simulink model "EST"  (R2026a)
settings: Solver=FixedStepAuto  StopTime=stopt  FixedStep=deltat  MaxStep=0.05
InitFcn:
  | clear all;
  | close all;
  | clc;
  | 
  | % add the data and script directories
  | addpath('data','scripts');
  | 
  | % load the constants (units)
  | constants;
  | 
  | % load the simulation parameters
  | preprocessing;
StopFcn:
  | postprocessing;
values from neighbouring files (symbols this model uses):
  alphaLoss = 0.15    [preprocessing.m]
  alphaSplit = 0.7    [preprocessing.m]
  areaTank = 6 * sideLength^2    (= 57.9293630763)    [preprocessing.m]
  cableArea = 6e-6    (= 6e-06)    [preprocessing.m]
  cableLength = 28.5    [preprocessing.m]
  cableLengthDemand = 20    [preprocessing.m]
  cableResistivity = 1.676e-8    (= 1.676e-08)    [preprocessing.m]
  cps = 920    [preprocessing.m]
  current = 20    [preprocessing.m]
  currentDemand = 2.5    [preprocessing.m]
  dh_ads = 2.5e6    (= 2500000)    [preprocessing.m]
  dtController = 900    [preprocessing.m]
  E = E_DA    (= 6000)    [preprocessing.m]
  EBatteryMax = 200 * 3.6e6    (= 720000000)    [preprocessing.m]
  EBatteryMin = 0  * 3.6e6    (= 0)    [preprocessing.m]
  efficiencyBatteryCharge = 0.95    [preprocessing.m]
  efficiencyInjection = 0.98    [preprocessing.m]
  emissivitySurface = 0.5    [preprocessing.m]
  emissivitySurfacePipe = 0.9    [preprocessing.m]
  EStorageMax = 5000 * 3.6e6    (= 18000000000)    [preprocessing.m]
  EStorageMin = 100  * 3.6e6    (= 360000000)    [preprocessing.m]
  etaBatteryDischarge = 0.95    [preprocessing.m]
  hAir = 10    [preprocessing.m]
  kInsulation = 0.04    [preprocessing.m]
  kLdf = 0.008    [preprocessing.m]
  kPipe = 0.3    [preprocessing.m]
  kSteel = 54    [preprocessing.m]
  mCpTotal = massGel * heatCapacityGel + massSteel * heatCapacitySteel    (= 21486379.4261)    [preprocessing.m]
  ms = massGel    (= 21600)    [preprocessing.m]
  n = 1.5    [preprocessing.m]
  pipeLength = 10    [preprocessing.m]
  PmaxBatteryCharge = 20    [preprocessing.m]
  PmaxBatteryDischarge = 20    [preprocessing.m]
  PmaxSorptionCharge = 5    [preprocessing.m]
  PmaxSorptionDischarge = 15    [preprocessing.m]
  pv = 1200    [preprocessing.m]
  r1 = 0.03    [preprocessing.m]
  r2 = 0.035    [preprocessing.m]
  r3 = 0.05    [preprocessing.m]
  stefanBoltz = 5.67e-8    (= 5.67e-08)    [preprocessing.m]
  tempEnv = 293.15    [preprocessing.m]
  Tfluid = 353.15    [preprocessing.m]
  thicknessInsulation = 0.10    (= 0.1)    [preprocessing.m]
  thicknessSteel = 0.015    [preprocessing.m]
  Tref = tempEnv    (= 293.15)    [preprocessing.m]
  TStorageInitial = Tref    (= 293.15)    [preprocessing.m]
  UA = 15    [preprocessing.m]
  X0 = 0.35    [preprocessing.m]
  Xref = X0    (= 0.35)    [preprocessing.m]
  XStorageInitial = max(0.0, min(X0, XStorageInitial))    [preprocessing.m]
settings Model: Creator=joche  LastModifiedBy=nimaaminpour
settings SimscapeCC: SimscapeLogDataHistory=5000.0  SimscapeNominalValues="[{\"value\":\"1\",\"unit\":\"A\"},{\"value\":\"1\",\"unit\":\"bar\"},{\"value\":\"1\",\"unit\":\"cm^2\"},{\"value\":\"1\",\"unit\":\"cm^3/s\"},{\"value\":\"1\",\"unit\":\"kJ/kg\"},{\"value\":\"1\",\"unit\":\"kW\"},{\"value\":\"1\",\"unit\":\"l\"},{\"value\":\"1\",\"unit\":\"N\"},{\"value\":\"1\",\"unit\":\"N*m\"},{\"value\":\"1\",\"unit\":\"V\"}]"  SimscapeLogType=none

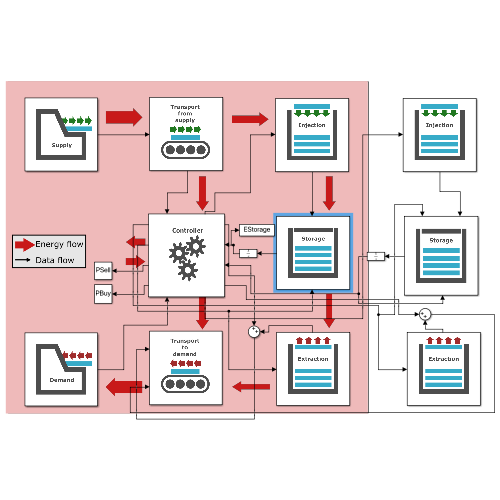
[thumbnail: Simulink's stored preview of the top-level diagram]
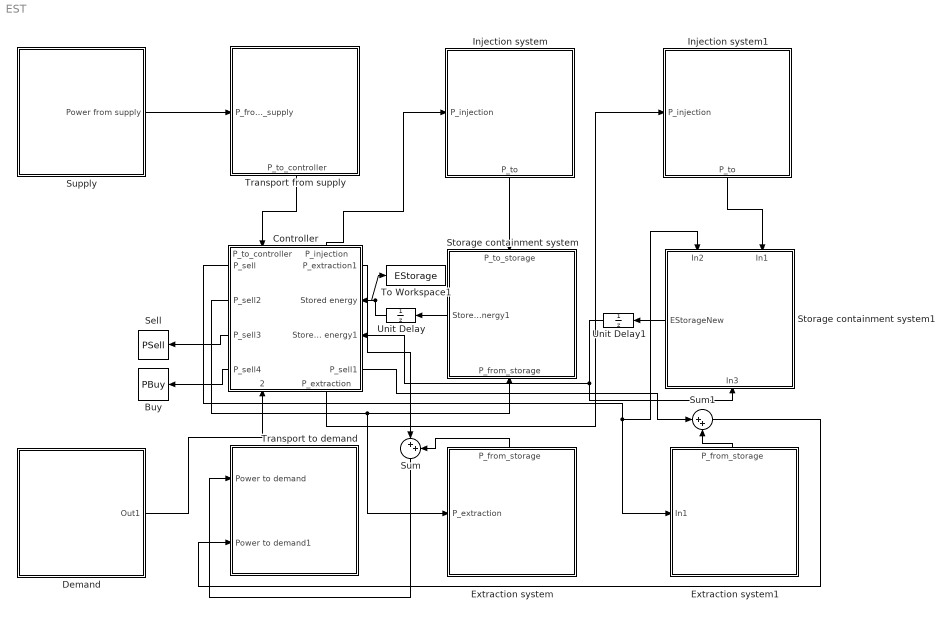
== system EST ==
  Buy : ToWorkspace  VariableName=PBuy  SampleTime=-1
  Controller : Subsystem
      settings: PortSchema="{\"entries\":[{\"content\":{\"sides\":[{\"content\":{\"connectorIds\":[\"Out5\",\"Out6\",\"Out7\",\"Out8\"]},\"type\":\"ConnectorPlacement.EquallySpacedRectSide\",\"uuid\":\"4daf33ce-c96a-4783-b5c4-228eed953e01\"},{\"content\":{\"connectorIds\":[\"Out1\",\"In3\",\"In4\",\"Out2\"],\"side\":\"RIGHT\"},\"type\":\"ConnectorPlacement.EquallySpacedRectSide\",\"uuid\":\"e9942e50-8467-4af8-b79b-80636cbc76e5\"},{\"content\":{\"connectorIds\":[\"In1\",\"Out4\"],\"side\":\"TOP\"},\"type\":\"ConnectorPlacement.EquallySpacedRectSide\",\"uuid\":\"f315e931-d69b-4751-b712-f89c6c81baeb\"},{\"content\":{\"connectorIds\":[\"In2\",\"Out3\"],\"side\":\"BOTTOM\"},\"type\":\"ConnectorPlacement.EquallySpacedRectSide\",\"uuid\":\"44715ee6-5cd5-4669-bcb9-5ed7c869bdb3\"}]},\"type\":\"ConnectorPlacement.EquallySpacedConnector\",\"uuid\":\"fff48899-944b-4064-b7d7-ecc12144fb48\"}],\"packageUris\":[\"http://schema.mathworks.com/mf0/Connector/R2020b\"],\"version\":\"1.0\"}"
      mask Display: image('$imagefile'); % Use "Edit Image" on toolstrip to change.
  Demand : Subsystem
      mask Display: image('$imagefile'); % Use "Edit Image" on toolstrip to change.
  Extraction system : Subsystem
      settings: PortSchema="{\"entries\":[{\"content\":{\"sides\":[{\"content\":{\"connectorIds\":[]},\"type\":\"ConnectorPlacement.EquallySpacedRectSide\",\"uuid\":\"05c5933d-55fc-4e06-853f-fc26d42905f9\"},{\"content\":{\"connectorIds\":[\"In1\"],\"side\":\"RIGHT\"},\"type\":\"ConnectorPlacement.EquallySpacedRectSide\",\"uuid\":\"327426c5-31d5-498b-a2bd-83e49353408c\"},{\"content\":{\"connectorIds\":[],\"side\":\"TOP\"},\"type\":\"ConnectorPlacement.EquallySpacedRectSide\",\"uuid\":\"55306cf3-a3de-4385-a5ae-b8600ecdd5a2\"},{\"content\":{\"connectorIds\":[\"Out1\"],\"side\":\"BOTTOM\"},\"type\":\"ConnectorPlacement.EquallySpacedRectSide\",\"uuid\":\"08fcc9c3-40d3-4ac6-b914-dfeef6039ffb\"}]},\"type\":\"ConnectorPlacement.EquallySpacedConnector\",\"uuid\":\"cb35d5ba-e8c6-462c-b7b2-fe8356d4b0a1\"}],\"packageUris\":[\"http://schema.mathworks.com/mf0/Connector/R2020b\"],\"version\":\"1.0\"}"
      mask Display: image('$imagefile'); % Use "Edit Image" on toolstrip to change.
  Extraction system1 : Subsystem
      settings: PortSchema="{\"entries\":[{\"content\":{\"sides\":[{\"content\":{},\"type\":\"ConnectorPlacement.EquallySpacedRectSide\",\"uuid\":\"05c5933d-55fc-4e06-853f-fc26d42905f9\"},{\"content\":{\"connectorIds\":[\"In1\"],\"side\":\"RIGHT\"},\"type\":\"ConnectorPlacement.EquallySpacedRectSide\",\"uuid\":\"327426c5-31d5-498b-a2bd-83e49353408c\"},{\"content\":{\"side\":\"TOP\"},\"type\":\"ConnectorPlacement.EquallySpacedRectSide\",\"uuid\":\"55306cf3-a3de-4385-a5ae-b8600ecdd5a2\"},{\"content\":{\"connectorIds\":[\"Out1\"],\"side\":\"BOTTOM\"},\"type\":\"ConnectorPlacement.EquallySpacedRectSide\",\"uuid\":\"08fcc9c3-40d3-4ac6-b914-dfeef6039ffb\"}]},\"type\":\"ConnectorPlacement.EquallySpacedConnector\",\"uuid\":\"cb35d5ba-e8c6-462c-b7b2-fe8356d4b0a1\"}],\"packageUris\":[\"http://schema.mathworks.com/mf0/Connector/R2020b\"],\"version\":\"1.0\"}"
      mask Display: image('$imagefile'); % Use "Edit Image" on toolstrip to change.
  Injection system : Subsystem
      settings: PortSchema="{\"entries\":[{\"content\":{\"sides\":[{\"content\":{\"connectorIds\":[]},\"type\":\"ConnectorPlacement.EquallySpacedRectSide\",\"uuid\":\"05c5933d-55fc-4e06-853f-fc26d42905f9\"},{\"content\":{\"connectorIds\":[\"In1\"],\"side\":\"RIGHT\"},\"type\":\"ConnectorPlacement.EquallySpacedRectSide\",\"uuid\":\"327426c5-31d5-498b-a2bd-83e49353408c\"},{\"content\":{\"connectorIds\":[\"Out1\"],\"side\":\"TOP\"},\"type\":\"ConnectorPlacement.EquallySpacedRectSide\",\"uuid\":\"55306cf3-a3de-4385-a5ae-b8600ecdd5a2\"},{\"content\":{\"connectorIds\":[],\"side\":\"BOTTOM\"},\"type\":\"ConnectorPlacement.EquallySpacedRectSide\",\"uuid\":\"08fcc9c3-40d3-4ac6-b914-dfeef6039ffb\"}]},\"type\":\"ConnectorPlacement.EquallySpacedConnector\",\"uuid\":\"cb35d5ba-e8c6-462c-b7b2-fe8356d4b0a1\"}],\"packageUris\":[\"http://schema.mathworks.com/mf0/Connector/R2020b\"],\"version\":\"1.0\"}"
      mask Display: image('$imagefile'); % Use "Edit Image" on toolstrip to change.
  Injection system1 : Subsystem
      settings: PortSchema="{\"entries\":[{\"content\":{\"sides\":[{\"content\":{\"connectorIds\":[]},\"type\":\"ConnectorPlacement.EquallySpacedRectSide\",\"uuid\":\"05c5933d-55fc-4e06-853f-fc26d42905f9\"},{\"content\":{\"connectorIds\":[\"In1\"],\"side\":\"RIGHT\"},\"type\":\"ConnectorPlacement.EquallySpacedRectSide\",\"uuid\":\"327426c5-31d5-498b-a2bd-83e49353408c\"},{\"content\":{\"connectorIds\":[\"Out1\"],\"side\":\"TOP\"},\"type\":\"ConnectorPlacement.EquallySpacedRectSide\",\"uuid\":\"55306cf3-a3de-4385-a5ae-b8600ecdd5a2\"},{\"content\":{\"connectorIds\":[],\"side\":\"BOTTOM\"},\"type\":\"ConnectorPlacement.EquallySpacedRectSide\",\"uuid\":\"08fcc9c3-40d3-4ac6-b914-dfeef6039ffb\"}]},\"type\":\"ConnectorPlacement.EquallySpacedConnector\",\"uuid\":\"cb35d5ba-e8c6-462c-b7b2-fe8356d4b0a1\"}],\"packageUris\":[\"http://schema.mathworks.com/mf0/Connector/R2020b\"],\"version\":\"1.0\"}"
      mask Display: image('$imagefile'); % Use "Edit Image" on toolstrip to change.
  Sell : ToWorkspace  VariableName=PSell  SampleTime=-1
  Storage containment system : Subsystem
      settings: PortSchema="{\"entries\":[{\"content\":{\"sides\":[{\"content\":{\"connectorIds\":[\"Out1\"]},\"type\":\"ConnectorPlacement.EquallySpacedRectSide\",\"uuid\":\"0ba48424-33b9-4934-970f-64fe5d8b070e\"},{\"content\":{\"connectorIds\":[],\"side\":\"RIGHT\"},\"type\":\"ConnectorPlacement.EquallySpacedRectSide\",\"uuid\":\"9cde340f-8f39-4499-9a12-5e1623737660\"},{\"content\":{\"connectorIds\":[\"In1\"],\"side\":\"TOP\"},\"type\":\"ConnectorPlacement.EquallySpacedRectSide\",\"uuid\":\"2af8db04-7fd0-4902-8637-8dc00edb4598\"},{\"content\":{\"connectorIds\":[\"In2\"],\"side\":\"BOTTOM\"},\"type\":\"ConnectorPlacement.EquallySpacedRectSide\",\"uuid\":\"e21ea806-d777-41a3-a53f-556fae66854b\"}]},\"type\":\"ConnectorPlacement.EquallySpacedConnector\",\"uuid\":\"4e2ddb36-4db3-4ab4-858b-ebb8ccefeb1f\"}],\"packageUris\":[\"http://schema.mathworks.com/mf0/Connector/R2020b\"],\"version\":\"1.0\"}"
      mask Display: image('$imagefile'); % Use "Edit Image" on toolstrip to change.
  Storage containment system1 : Subsystem
      settings: PortSchema="{\"entries\":[{\"content\":{\"sides\":[{\"content\":{\"connectorIds\":[\"Out1\"]},\"type\":\"ConnectorPlacement.EquallySpacedRectSide\",\"uuid\":\"0ba48424-33b9-4934-970f-64fe5d8b070e\"},{\"content\":{\"side\":\"RIGHT\"},\"type\":\"ConnectorPlacement.EquallySpacedRectSide\",\"uuid\":\"9cde340f-8f39-4499-9a12-5e1623737660\"},{\"content\":{\"connectorIds\":[\"In1\",\"In2\"],\"side\":\"TOP\"},\"type\":\"ConnectorPlacement.EquallySpacedRectSide\",\"uuid\":\"2af8db04-7fd0-4902-8637-8dc00edb4598\"},{\"content\":{\"connectorIds\":[\"In3\"],\"side\":\"BOTTOM\"},\"type\":\"ConnectorPlacement.EquallySpacedRectSide\",\"uuid\":\"e21ea806-d777-41a3-a53f-556fae66854b\"}]},\"type\":\"ConnectorPlacement.EquallySpacedConnector\",\"uuid\":\"4e2ddb36-4db3-4ab4-858b-ebb8ccefeb1f\"}],\"packageUris\":[\"http://schema.mathworks.com/mf0/Connector/R2020b\"],\"version\":\"1.0\"}"
      mask Display: image('$imagefile'); % Use "Edit Image" on toolstrip to change.
  Sum : Sum  Inputs=|++
  Sum1 : Sum  Inputs=|++
  Supply : Subsystem
      mask Display: image('$imagefile'); % Use "Edit Image" on toolstrip to change.
  To Workspace1 : ToWorkspace  VariableName=EStorage  SampleTime=-1
  Transport from supply : Subsystem
      settings: PortSchema="{\"entries\":[{\"content\":{\"sides\":[{\"content\":{\"connectorIds\":[\"In1\"]},\"type\":\"ConnectorPlacement.EquallySpacedRectSide\",\"uuid\":\"31329006-3d36-4d93-9c44-7503a515d397\"},{\"content\":{\"connectorIds\":[],\"side\":\"RIGHT\"},\"type\":\"ConnectorPlacement.EquallySpacedRectSide\",\"uuid\":\"aba139c7-f9b6-4881-a56b-a4cbbedacd88\"},{\"content\":{\"connectorIds\":[],\"side\":\"TOP\"},\"type\":\"ConnectorPlacement.EquallySpacedRectSide\",\"uuid\":\"e683eb73-7a35-4160-9c39-da83856a6278\"},{\"content\":{\"connectorIds\":[\"Out1\"],\"side\":\"BOTTOM\"},\"type\":\"ConnectorPlacement.EquallySpacedRectSide\",\"uuid\":\"1170dd18-447c-437f-9043-6812c2877331\"}]},\"type\":\"ConnectorPlacement.EquallySpacedConnector\",\"uuid\":\"804af608-1d70-444f-af69-e05f19bf98f3\"}],\"packageUris\":[\"http://schema.mathworks.com/mf0/Connector/R2020b\"],\"version\":\"1.0\"}"
      mask Display: image('$imagefile'); % Use "Edit Image" on toolstrip to change.
  Transport to demand : Subsystem
      mask Display: image('$imagefile'); % Use "Edit Image" on toolstrip to change.
  Unit Delay : UnitDelay  SampleTime=-1
  Unit Delay1 : UnitDelay  SampleTime=-1
  wires:
  Supply/1(Power from supply) -> Transport from supply/1(P_from_supply)
  Transport from supply/1(P_to_controller) -> Controller/1(P_to_controller)
  Injection system/1(P_to) -> Storage containment system/1(P_to_storage)
  Storage containment system/1(Stored energy1) -> Unit Delay/1
  Controller/8(P_sell4) -> Buy/1
  Injection system1/1(P_to) -> Storage containment system1/2(In1)
  Storage containment system1/1(EStorageNew) -> Unit Delay1/1
  Demand/1(Out1) -> Controller/2(P_from_controller)
  Unit Delay/1 -> To Workspace1/1, Controller/3(Stored energy)
  Unit Delay1/1 -> Storage containment system1/3(In3), Controller/4(Stored energy1)
  Controller/7(P_sell3) -> Sell/1
  Controller/5(P_sell) -> Storage containment system1/1(In2), Extraction system1/1(In1)
  Controller/6(P_sell2) -> Storage containment system/2(P_from_storage), Extraction system/1(P_extraction)
  Controller/1(P_extraction1) -> Sum/1
  Extraction system/1(P_from_storage) -> Sum/2
  Controller/2(P_sell1) -> Sum1/1
  Extraction system1/1(P_from_storage) -> Sum1/2
  Sum/1 -> Transport to demand/1(Power to demand)
  Sum1/1 -> Transport to demand/2(Power to demand1)
  Controller/3(P_extraction) -> Injection system1/1(P_injection)
  Controller/4(P_injection) -> Injection system/1(P_injection)

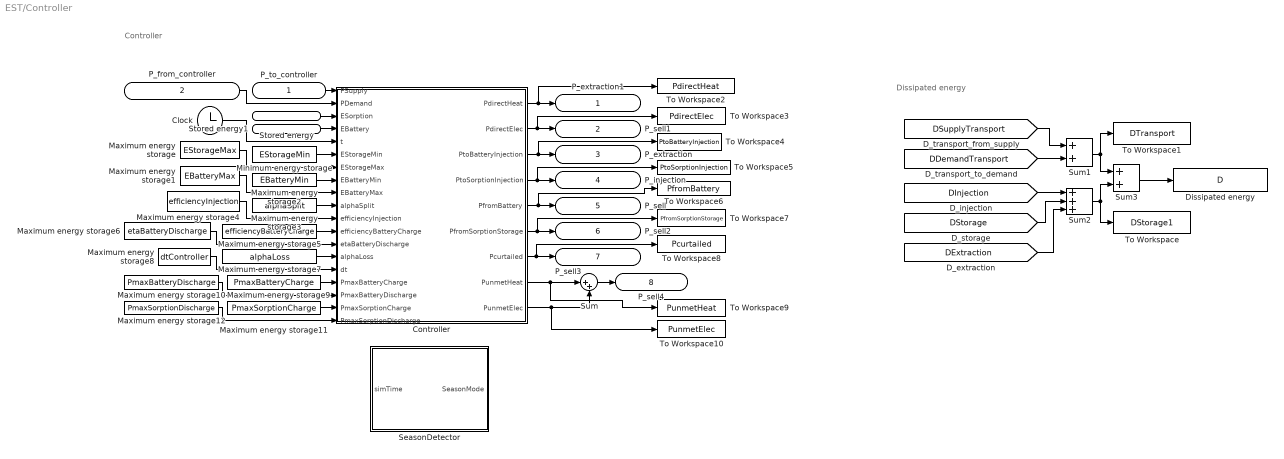
== system EST/Controller ==
  note: Dissipated energy
  note: Controller
  P_to_controller : Inport
  P_from_controller : Inport  Port=2
  Stored energy : Inport  Port=3
  Stored energy1 : Inport  Port=4
  Clock : Clock
  Controller : MATLAB Function  TreatAsAtomicUnit=on
  Dissipated energy : ToWorkspace  VariableName=D  SampleTime=-1
  Maximum energy storage : Constant  Value=EStorageMax
  Maximum energy storage1 : Constant  Value=EBatteryMax
  Maximum energy storage10 : Constant  Value=PmaxBatteryDischarge
  Maximum energy storage11 : Constant  Value=PmaxSorptionCharge
  Maximum energy storage12 : Constant  Value=PmaxSorptionDischarge
  Maximum energy storage2 : Constant  Value=EBatteryMin
  Maximum energy storage3 : Constant  Value=alphaSplit
  Maximum energy storage4 : Constant  Value=efficiencyInjection
  Maximum energy storage5 : Constant  Value=efficiencyBatteryCharge
  Maximum energy storage6 : Constant  Value=etaBatteryDischarge
  Maximum energy storage7 : Constant  Value=alphaLoss
  Maximum energy storage8 : Constant  Value=dtController
  Maximum energy storage9 : Constant  Value=PmaxBatteryCharge
  Minimum energy storage : Constant  Value=EStorageMin
  SeasonDetector : MATLAB Function  TreatAsAtomicUnit=on
  Sum : Sum  Inputs=|++
  Sum1 : Sum
  Sum2 : Sum  Inputs=+++
  Sum3 : Sum
  To Workspace : ToWorkspace  VariableName=DStorage1  SampleTime=-1
  To Workspace1 : ToWorkspace  VariableName=DTransport  SampleTime=-1
  To Workspace10 : ToWorkspace  VariableName=PunmetElec  SampleTime=-1
  To Workspace2 : ToWorkspace  VariableName=PdirectHeat  SampleTime=-1
  To Workspace3 : ToWorkspace  VariableName=PdirectElec  SampleTime=-1
  To Workspace4 : ToWorkspace  VariableName=PtoBatteryInjection  SampleTime=-1
  To Workspace5 : ToWorkspace  VariableName=PtoSorptionInjection  SampleTime=-1
  To Workspace6 : ToWorkspace  VariableName=PfromBattery  SampleTime=-1
  To Workspace7 : ToWorkspace  VariableName=PfromSorptionStorage  SampleTime=-1
  To Workspace8 : ToWorkspace  VariableName=Pcurtailed  SampleTime=-1
  To Workspace9 : ToWorkspace  VariableName=PunmetHeat  SampleTime=-1
  P_extraction1 : Outport
  P_sell1 : Outport  Port=2
  P_extraction : Outport  Port=3
  P_injection : Outport  Port=4
  P_sell : Outport  Port=5
  P_sell2 : Outport  Port=6
  P_sell3 : Outport  Port=7
  P_sell4 : Outport  Port=8
  wires:
  [DDemandTransport] -> Sum1/2
  [DSupplyTransport] -> Sum1/1
  [DInjection] -> Sum2/1
  [DStorage] -> Sum2/2
  [DExtraction] -> Sum2/3
  Sum2/1 -> To Workspace/1, Sum3/2
  Sum1/1 -> To Workspace1/1, Sum3/1
  Sum3/1 -> Dissipated energy/1
  P_to_controller/1 -> Controller/1(PSupply)
  P_from_controller/1 -> Controller/2(PDemand)
  Stored energy/1 -> Controller/3(ESorption)
  Stored energy1/1 -> Controller/4(EBattery)
  Clock/1 -> Controller/5(t)
  Maximum energy storage2/1 -> Controller/8(EBatteryMin)
  Minimum energy storage/1 -> Controller/6(EStorageMin)
  Maximum energy storage/1 -> Controller/7(EStorageMax)
  Maximum energy storage1/1 -> Controller/9(EBatteryMax)
  Maximum energy storage3/1 -> Controller/10(alphaSplit)
  Maximum energy storage4/1 -> Controller/11(efficiencyInjection)
  Maximum energy storage5/1 -> Controller/12(efficiencyBatteryCharge)
  Maximum energy storage6/1 -> Controller/13(etaBatteryDischarge)
  Maximum energy storage7/1 -> Controller/14(alphaLoss)
  Maximum energy storage8/1 -> Controller/15(dt)
  Maximum energy storage9/1 -> Controller/16(PmaxBatteryCharge)
  Maximum energy storage10/1 -> Controller/17(PmaxBatteryDischarge)
  Maximum energy storage11/1 -> Controller/18(PmaxSorptionCharge)
  Maximum energy storage12/1 -> Controller/19(PmaxSorptionDischarge)
  Controller/1(PdirectHeat) -> P_extraction1/1, To Workspace2/1
  Controller/2(PdirectElec) -> P_sell1/1, To Workspace3/1
  Controller/3(PtoBatteryInjection) -> To Workspace4/1, P_extraction/1
  Controller/4(PtoSorptionInjection) -> P_injection/1, To Workspace5/1
  Controller/5(PfromBattery) -> To Workspace6/1, P_sell/1
  Controller/6(PfromSorptionStorage) -> To Workspace7/1, P_sell2/1
  Controller/7(Pcurtailed) -> To Workspace8/1, P_sell3/1
  Controller/8(PunmetHeat) -> To Workspace9/1, Sum/1
  Controller/9(PunmetElec) -> To Workspace10/1, Sum/2
  Sum/1 -> P_sell4/1

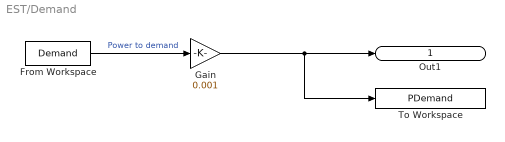
== system EST/Demand ==
  From Workspace : FromWorkspace  VariableName=Demand  OutputAfterFinalValue=Setting to zero
  Gain : Gain  Gain=0.001
  To Workspace : ToWorkspace  VariableName=PDemand  SampleTime=-1
  Out1 : Outport
  wires:
  From Workspace/1 -> Gain/1  "Power to demand"
  Gain/1 -> To Workspace/1, Out1/1

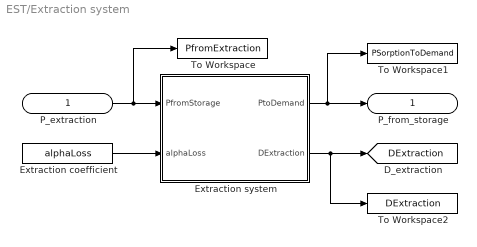
== system EST/Extraction system ==
  P_extraction : Inport
  Extraction coefficient : Constant  Value=alphaLoss
  Extraction system : MATLAB Function  TreatAsAtomicUnit=on
  To Workspace : ToWorkspace  VariableName=PfromExtraction  SampleTime=-1
  To Workspace1 : ToWorkspace  VariableName=PSorptionToDemand  SampleTime=-1
  To Workspace2 : ToWorkspace  VariableName=DExtraction  SampleTime=-1
  P_from_storage : Outport
  tag scope: DExtraction=global
  wires:
  P_extraction/1 -> To Workspace/1, Extraction system/1(PfromStorage)
  Extraction system/1(PtoDemand) -> To Workspace1/1, P_from_storage/1
  Extraction system/2(DExtraction) -> To Workspace2/1, [DExtraction]
  Extraction coefficient/1 -> Extraction system/2(alphaLoss)

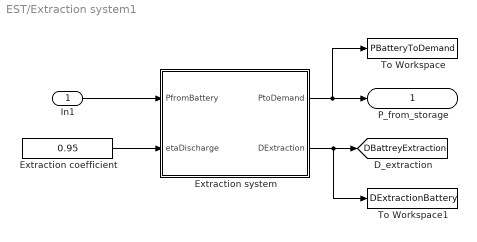
== system EST/Extraction system1 ==
  In1 : Inport
  Extraction coefficient : Constant  Value=0.95
  Extraction system : MATLAB Function  TreatAsAtomicUnit=on
  To Workspace : ToWorkspace  VariableName=PBatteryToDemand  SampleTime=-1
  To Workspace1 : ToWorkspace  VariableName=DExtractionBattery  SampleTime=-1
  P_from_storage : Outport
  tag scope: DBattreyExtraction=global
  wires:
  In1/1 -> Extraction system/1(PfromBattery)
  Extraction system/1(PtoDemand) -> To Workspace/1, P_from_storage/1
  Extraction system/2(DExtraction) -> To Workspace1/1, [DBattreyExtraction]
  Extraction coefficient/1 -> Extraction system/2(etaDischarge)

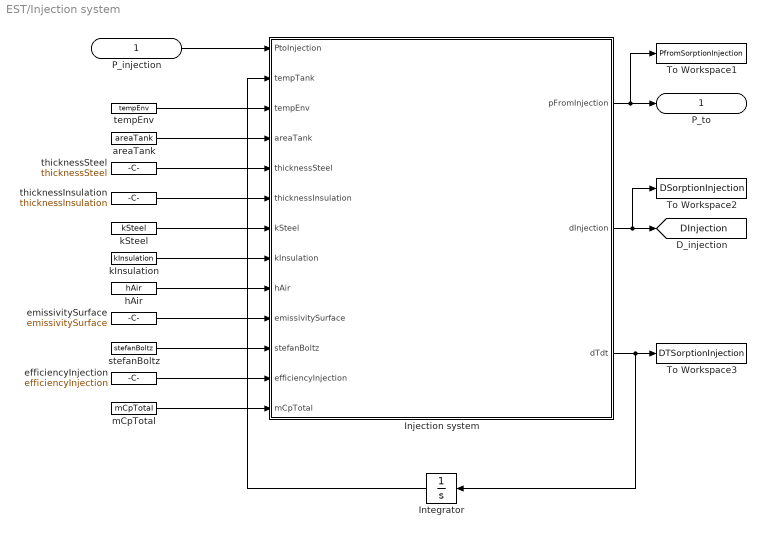
== system EST/Injection system ==
  P_injection : Inport
  Injection system : MATLAB Function  TreatAsAtomicUnit=on
  Integrator : Integrator  InitialCondition=293.15
  To Workspace1 : ToWorkspace  VariableName=PfromSorptionInjection  SampleTime=-1
  To Workspace2 : ToWorkspace  VariableName=DSorptionInjection  SampleTime=-1
  To Workspace3 : ToWorkspace  VariableName=DTSorptionInjection  SampleTime=-1
  areaTank : Constant  Value=areaTank
  efficiencyInjection : Constant  Value=efficiencyInjection
  emissivitySurface : Constant  Value=emissivitySurface
  hAir : Constant  Value=hAir
  kInsulation : Constant  Value=kInsulation
  kSteel : Constant  Value=kSteel
  mCpTotal : Constant  Value=mCpTotal
  stefanBoltz : Constant  Value=stefanBoltz
  tempEnv : Constant  Value=tempEnv
  thicknessInsulation : Constant  Value=thicknessInsulation
  thicknessSteel : Constant  Value=thicknessSteel
  P_to : Outport
  tag scope: DInjection=global
  wires:
  P_injection/1 -> Injection system/1(PtoInjection)
  Injection system/1(pFromInjection) -> To Workspace1/1, P_to/1
  Injection system/2(dInjection) -> To Workspace2/1, [DInjection]
  Injection system/3(dTdt) -> To Workspace3/1, Integrator/1
  Integrator/1 -> Injection system/2(tempTank)
  tempEnv/1 -> Injection system/3(tempEnv)
  areaTank/1 -> Injection system/4(areaTank)
  thicknessSteel/1 -> Injection system/5(thicknessSteel)
  thicknessInsulation/1 -> Injection system/6(thicknessInsulation)
  kSteel/1 -> Injection system/7(kSteel)
  kInsulation/1 -> Injection system/8(kInsulation)
  hAir/1 -> Injection system/9(hAir)
  emissivitySurface/1 -> Injection system/10(emissivitySurface)
  stefanBoltz/1 -> Injection system/11(stefanBoltz)
  efficiencyInjection/1 -> Injection system/12(efficiencyInjection)
  mCpTotal/1 -> Injection system/13(mCpTotal)

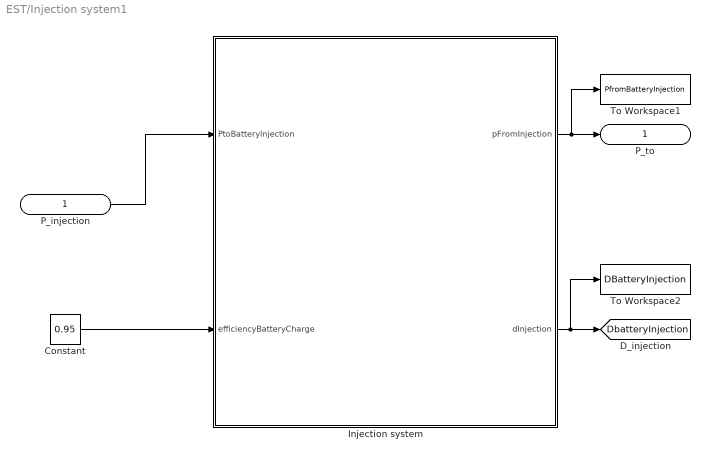
== system EST/Injection system1 ==
  P_injection : Inport
  Constant : Constant  Value=0.95
  Injection system : MATLAB Function  TreatAsAtomicUnit=on
  To Workspace1 : ToWorkspace  VariableName=PfromBatteryInjection  SampleTime=-1
  To Workspace2 : ToWorkspace  VariableName=DBatteryInjection  SampleTime=-1
  P_to : Outport
  tag scope: DbatteryInjection=global
  wires:
  P_injection/1 -> Injection system/1(PtoBatteryInjection)
  Injection system/1(pFromInjection) -> To Workspace1/1, P_to/1
  Injection system/2(dInjection) -> To Workspace2/1, [DbatteryInjection]
  Constant/1 -> Injection system/2(efficiencyBatteryCharge)

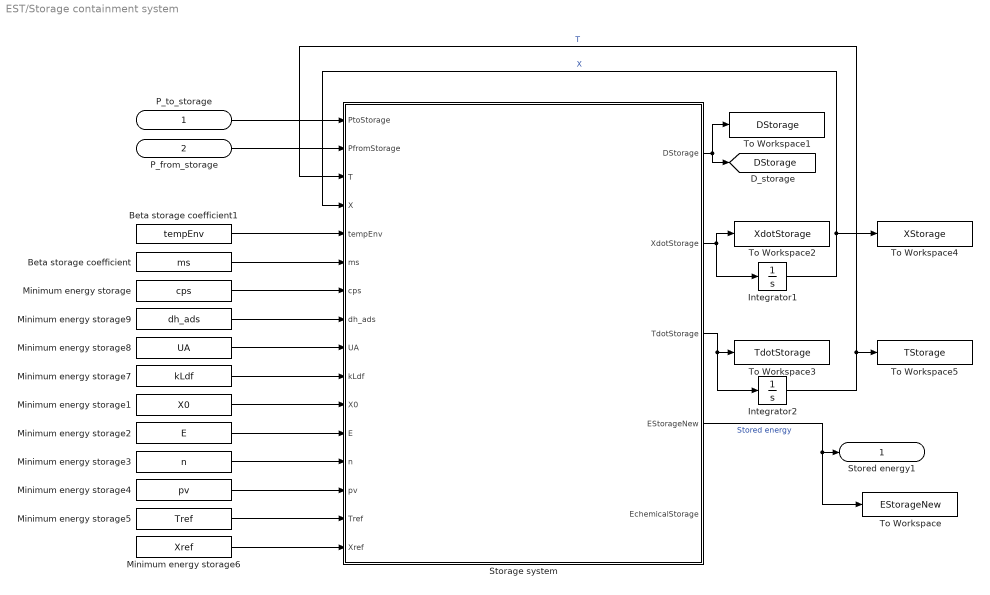
== system EST/Storage containment system ==
  P_to_storage : Inport
  P_from_storage : Inport  Port=2
  Beta storage coefficient : Constant  Value=ms
  Beta storage coefficient1 : Constant  Value=tempEnv
  Integrator1 : Integrator  InitialCondition=XStorageInitial
  Integrator2 : Integrator  InitialCondition=TStorageInitial
  Minimum energy storage : Constant  Value=cps
  Minimum energy storage1 : Constant  Value=X0
  Minimum energy storage2 : Constant  Value=E
  Minimum energy storage3 : Constant  Value=n
  Minimum energy storage4 : Constant  Value=pv
  Minimum energy storage5 : Constant  Value=Tref
  Minimum energy storage6 : Constant  Value=Xref
  Minimum energy storage7 : Constant  Value=kLdf
  Minimum energy storage8 : Constant  Value=UA
  Minimum energy storage9 : Constant  Value=dh_ads
  Storage system : MATLAB Function  TreatAsAtomicUnit=on
  To Workspace : ToWorkspace  VariableName=EStorageNew  SampleTime=-1
  To Workspace1 : ToWorkspace  VariableName=DStorage  SampleTime=-1
  To Workspace2 : ToWorkspace  VariableName=XdotStorage  SampleTime=-1
  To Workspace3 : ToWorkspace  VariableName=TdotStorage  SampleTime=-1
  To Workspace4 : ToWorkspace  VariableName=XStorage  SampleTime=-1
  To Workspace5 : ToWorkspace  VariableName=TStorage  SampleTime=-1
  Stored energy1 : Outport
  tag scope: DStorage=global
  wires:
  P_from_storage/1 -> Storage system/2(PfromStorage)
  P_to_storage/1 -> Storage system/1(PtoStorage)
  Storage system/4(EStorageNew) -> To Workspace/1, Stored energy1/1  "Stored energy"
  Storage system/1(DStorage) -> [DStorage], To Workspace1/1
  Beta storage coefficient/1 -> Storage system/6(ms)
  Minimum energy storage/1 -> Storage system/7(cps)
  Minimum energy storage1/1 -> Storage system/11(X0)
  Minimum energy storage2/1 -> Storage system/12(E)
  Minimum energy storage3/1 -> Storage system/13(n)
  Minimum energy storage4/1 -> Storage system/14(pv)
  Minimum energy storage7/1 -> Storage system/10(kLdf)
  Minimum energy storage8/1 -> Storage system/9(UA)
  Beta storage coefficient1/1 -> Storage system/5(tempEnv)
  Minimum energy storage9/1 -> Storage system/8(dh_ads)
  Storage system/2(XdotStorage) -> Integrator1/1, To Workspace2/1
  Integrator1/1 -> Storage system/4(X), To Workspace4/1  "X"
  Storage system/3(TdotStorage) -> Integrator2/1, To Workspace3/1
  Integrator2/1 -> Storage system/3(T), To Workspace5/1  "T"
  Minimum energy storage5/1 -> Storage system/15(Tref)
  Minimum energy storage6/1 -> Storage system/16(Xref)

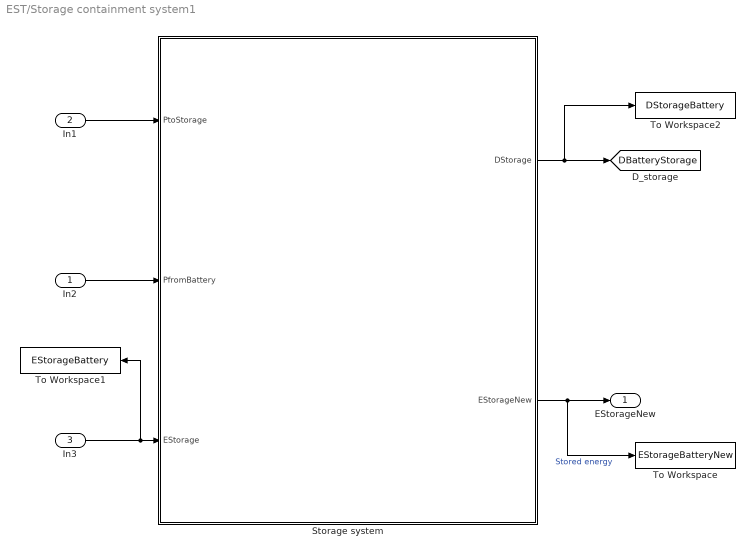
== system EST/Storage containment system1 ==
  In2 : Inport
  In1 : Inport  Port=2
  In3 : Inport  Port=3
  Storage system : MATLAB Function  TreatAsAtomicUnit=on
  To Workspace : ToWorkspace  VariableName=EStorageBatteryNew  SampleTime=-1
  To Workspace1 : ToWorkspace  VariableName=EStorageBattery  SampleTime=-1
  To Workspace2 : ToWorkspace  VariableName=DStorageBattery  SampleTime=-1
  EStorageNew : Outport
  tag scope: DBatteryStorage=global
  wires:
  In2/1 -> Storage system/2(PfromBattery)
  In1/1 -> Storage system/1(PtoStorage)
  Storage system/2(EStorageNew) -> EStorageNew/1, To Workspace/1  "Stored energy"
  Storage system/1(DStorage) -> To Workspace2/1, [DBatteryStorage]
  In3/1 -> To Workspace1/1, Storage system/3(EStorage)

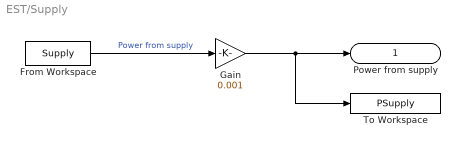
== system EST/Supply ==
  From Workspace : FromWorkspace  VariableName=Supply  OutputAfterFinalValue=Setting to zero
  Gain : Gain  Gain=0.001
  To Workspace : ToWorkspace  VariableName=PSupply  SampleTime=-1
  Power from supply : Outport
  wires:
  From Workspace/1 -> Gain/1  "Power from supply"
  Gain/1 -> To Workspace/1, Power from supply/1

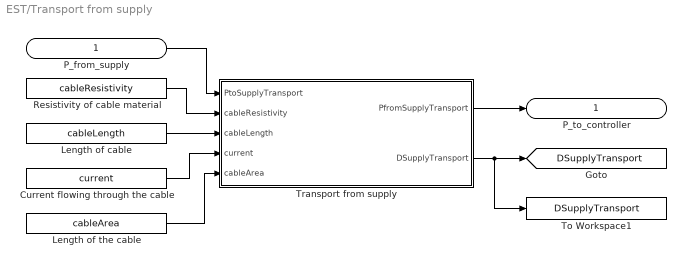
== system EST/Transport from supply ==
  P_from_supply : Inport
  Current flowing through the cable : Constant  Value=current
  Length of cable : Constant  Value=cableLength
  Length of the cable : Constant  Value=cableArea
  Resistivity of cable material : Constant  Value=cableResistivity
  To Workspace1 : ToWorkspace  VariableName=DSupplyTransport  SampleTime=-1
  Transport from supply : MATLAB Function  TreatAsAtomicUnit=on
  P_to_controller : Outport
  tag scope: DSupplyTransport=global
  wires:
  Transport from supply/1(PfromSupplyTransport) -> P_to_controller/1
  Transport from supply/2(DSupplyTransport) -> To Workspace1/1, [DSupplyTransport]
  P_from_supply/1 -> Transport from supply/1(PtoSupplyTransport)
  Resistivity of cable material/1 -> Transport from supply/2(cableResistivity)
  Current flowing through the cable/1 -> Transport from supply/4(current)
  Length of the cable/1 -> Transport from supply/5(cableArea)
  Length of cable/1 -> Transport from supply/3(cableLength)

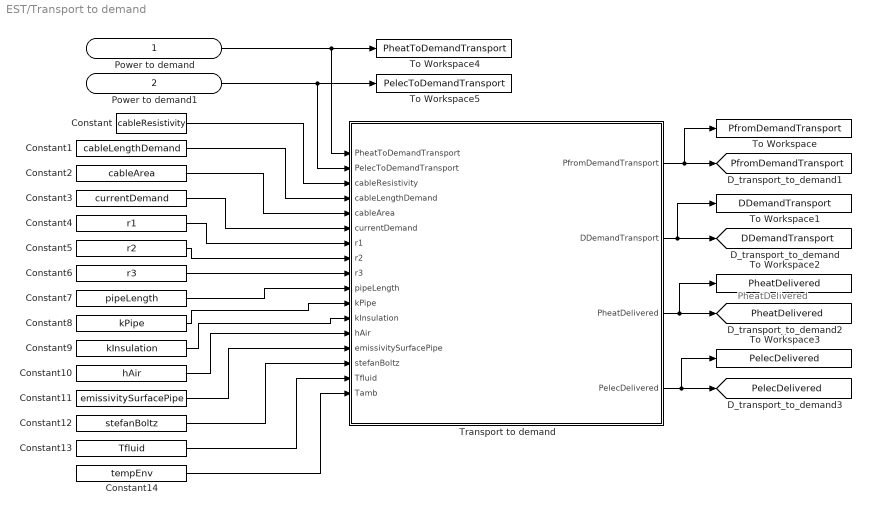
== system EST/Transport to demand ==
  note: PheatDelivered
  Power to demand : Inport
  Power to demand1 : Inport  Port=2
  Constant : Constant  Value=cableResistivity
  Constant1 : Constant  Value=cableLengthDemand
  Constant10 : Constant  Value=hAir
  Constant11 : Constant  Value=emissivitySurfacePipe
  Constant12 : Constant  Value=stefanBoltz
  Constant13 : Constant  Value=Tfluid
  Constant14 : Constant  Value=tempEnv
  Constant2 : Constant  Value=cableArea
  Constant3 : Constant  Value=currentDemand
  Constant4 : Constant  Value=r1
  Constant5 : Constant  Value=r2
  Constant6 : Constant  Value=r3
  Constant7 : Constant  Value=pipeLength
  Constant8 : Constant  Value=kPipe
  Constant9 : Constant  Value=kInsulation
  To Workspace : ToWorkspace  VariableName=PfromDemandTransport  SampleTime=-1
  To Workspace1 : ToWorkspace  VariableName=DDemandTransport  SampleTime=-1
  To Workspace2 : ToWorkspace  VariableName=PheatDelivered  SampleTime=-1
  To Workspace3 : ToWorkspace  VariableName=PelecDelivered  SampleTime=-1
  To Workspace4 : ToWorkspace  VariableName=PheatToDemandTransport  SampleTime=-1
  To Workspace5 : ToWorkspace  VariableName=PelecToDemandTransport  SampleTime=-1
  Transport to demand : MATLAB Function  TreatAsAtomicUnit=on
  tag scope: DDemandTransport=global, PelecDelivered=global, PfromDemandTransport=global, PheatDelivered=global
  wires:
  Power to demand1/1 -> Transport to demand/2(PelecToDemandTransport), To Workspace5/1
  Power to demand/1 -> Transport to demand/1(PheatToDemandTransport), To Workspace4/1
  Transport to demand/1(PfromDemandTransport) -> [PfromDemandTransport], To Workspace/1
  Transport to demand/2(DDemandTransport) -> To Workspace1/1, [DDemandTransport]
  Constant/1 -> Transport to demand/3(cableResistivity)
  Constant1/1 -> Transport to demand/4(cableLengthDemand)
  Constant2/1 -> Transport to demand/5(cableArea)
  Constant3/1 -> Transport to demand/6(currentDemand)
  Constant4/1 -> Transport to demand/7(r1)
  Constant5/1 -> Transport to demand/8(r2)
  Constant6/1 -> Transport to demand/9(r3)
  Constant7/1 -> Transport to demand/10(pipeLength)
  Constant8/1 -> Transport to demand/11(kPipe)
  Constant9/1 -> Transport to demand/12(kInsulation)
  Constant10/1 -> Transport to demand/13(hAir)
  Constant11/1 -> Transport to demand/14(emissivitySurfacePipe)
  Constant12/1 -> Transport to demand/15(stefanBoltz)
  Constant13/1 -> Transport to demand/16(Tfluid)
  Constant14/1 -> Transport to demand/17(Tamb)
  Transport to demand/3(PheatDelivered) -> To Workspace2/1, [PheatDelivered]
  Transport to demand/4(PelecDelivered) -> To Workspace3/1, [PelecDelivered]

== matlab function EST/Extraction system/Extraction system ==
  data: PfromStorage input; PtoDemand output; DExtraction output; alphaLoss input
function [PtoDemand, DExtraction] = extraction(PfromStorage, alphaLoss)

% Sorption Extraction subsystem
% Inputs and outputs are in kW.

PfromStorage = max(0.0, PfromStorage);

alphaLoss = max(0.0, min(1.0, alphaLoss));

DExtraction = alphaLoss * PfromStorage;
PtoDemand   = PfromStorage - DExtraction;

end

== matlab function EST/Storage containment system/Storage system ==
  data: DStorage output; PtoStorage input; PfromStorage input; T input; X input; tempEnv input; ms input; cps input; dh_ads input; UA input; XdotStorage output; TdotStorage output; kLdf input; X0 input; E input; n input; pv input; Tref input; Xref input; EStorageNew output; EchemicalStorage output
function [DStorage, XdotStorage, TdotStorage, EStorageNew, EchemicalStorage] = Storage(PtoStorage, PfromStorage, T, X, tempEnv, ms, cps, dh_ads, UA, kLdf, X0, E, n, pv, Tref, Xref)

% Sorption Storage subsystem
% PtoStorage and PfromStorage are in kW.
% Internal heat terms are in W.
% EStorageNew is in J.

R = 8.314; % [J/(mol*K)]
epsilon = 1e-9;

% Convert kW to W
PtoStorageW   = max(0.0, PtoStorage)   * 1000.0;
PfromStorageW = max(0.0, PfromStorage) * 1000.0;

% Safe values
T_safe       = max(T, 273.15);
tempEnv_safe = max(tempEnv, 1.0);

X0_safe = max(X0, epsilon);
X_safe  = max(0.0, min(X0_safe, X));

Xref_safe = max(0.0, min(X0_safe, Xref));

% Antoine equation for water saturation pressure
T_C = T_safe - 273.15;

A = 8.07131;
B = 1730.63;
C_antoine = 233.426;

C_denom = C_antoine + T_C;
if abs(C_denom) < 1e-4
    C_denom = 1e-4;
end

Psat_mmHg = 10^(A - B / C_denom);
psat      = max(Psat_mmHg * 133.322, epsilon);
pv_safe   = max(pv, epsilon);

% Dubinin-Astakhov equilibrium
ratio = max(psat / pv_safe, 1.0 + epsilon);

E_DA_safe = max(E, epsilon);
n_safe    = max(n, epsilon);

da_arg     = (R * T_safe / E_DA_safe) * log(ratio);
da_base    = max(0.0, da_arg);
da_exp_arg = max(-500.0, -(da_base ^ n_safe));

Xeq = X0_safe * exp(da_exp_arg);
Xeq = max(0.0, min(X0_safe, Xeq));

% Linear driving force kinetics
% IMPORTANT: Keep this original logic. Do not force Xdot based on charging mode.
kLdf_safe = max(kLdf, 0.0);

XdotStorage_raw = kLdf_safe * (Xeq - X_safe);
XdotStorage     = max(-0.01, min(0.01, XdotStorage_raw)); % [kg/kg/s]

% Heat terms
ms_safe  = max(ms, epsilon);
cps_safe = max(cps, epsilon);
UA_safe  = max(UA, 0.0);

% Positive Xdot = adsorption = heat released
% Negative Xdot = desorption = heat consumed
Qreaction = ms_safe * dh_ads * XdotStorage; % [W]

% Heat loss to environment
Qloss = UA_safe * (T_safe - tempEnv_safe); % [W]

% Temperature derivative
thermal_mass = ms_safe * cps_safe; % [J/K]

Tdot_num = PtoStorageW - PfromStorageW + Qreaction - Qloss;

TdotStorage_raw = Tdot_num / thermal_mass;
TdotStorage     = max(-5.0, min(5.0, TdotStorage_raw)); % [K/s]

% Stored energy
% Empty state should normally be wet/loaded sorbent: X = Xref = X0.

Echemical = ms_safe * dh_ads * (Xref_safe - X_safe);
Ethermal  = thermal_mass * (T_safe - Tref);

% Total stored energy, including sensible heat
EStorageNew = max(0.0, Echemical + Ethermal);

% Seasonal sorption storage state only
EchemicalStorage = max(0.0, Echemical);

% Storage dissipation in kW
DStorage = max(0.0, Qloss) / 1000.0;

end

== matlab function EST/Controller/SeasonDetector ==
  settings: updateMethod=DISCRETE
  data: SeasonMode output; simTime input
function SeasonMode = SeasonDetector(simTime)

dayOfYear = floor(simTime/86400) + 1;

% Summer: April to September
if dayOfYear >= 91 && dayOfYear <= 273
    SeasonMode = 1;   % Summer
else
    SeasonMode = 0;   % Winter
end

end

== matlab function EST/Transport to demand/Transport to demand ==
  data: PheatToDemandTransport input; PfromDemandTransport output; PelecToDemandTransport input; DDemandTransport output; cableResistivity input; cableLengthDemand input; cableArea input; currentDemand input; r1 input; r2 input; r3 input; pipeLength input; kPipe input; kInsulation input; hAir input; emissivitySurfacePipe input; stefanBoltz input; Tfluid input; Tamb input; PheatDelivered output; PelecDelivered output
function [PfromDemandTransport, DDemandTransport, PheatDelivered, PelecDelivered] = demandTransport(PheatToDemandTransport, PelecToDemandTransport, cableResistivity, cableLengthDemand, cableArea, currentDemand, r1, r2, r3, pipeLength, kPipe, kInsulation, hAir, emissivitySurfacePipe, stefanBoltz, Tfluid, Tamb)

epsilon = 1e-9;

PheatToDemandTransport = max(0.0, PheatToDemandTransport);
PelecToDemandTransport = max(0.0, PelecToDemandTransport);

% ELECTRICAL TRANSPORT
cableArea_safe = max(cableArea, epsilon);
R = cableResistivity * (2.0 * cableLengthDemand / cableArea_safe);

PlossElec = (currentDemand^2 * R) / 1000.0; % [kW]

PelecDelivered = max(0.0, PelecToDemandTransport - PlossElec);

% THERMAL TRANSPORT
Tfluid_safe = max(Tfluid, 1.0);
Tamb_safe   = max(Tamb,   1.0);

r1_safe = max(r1, epsilon);
r2_safe = max(r2, 2.0 * r1_safe);
r3_safe = max(r3, 2.0 * r2_safe);

kPipe_safe       = max(kPipe,       epsilon);
kInsulation_safe = max(kInsulation, epsilon);
pipeLength_safe  = max(pipeLength,  epsilon);

Rcond = log(r2_safe / r1_safe) / (2.0 * pi * kPipe_safe * pipeLength_safe) ...
    + log(r3_safe / r2_safe) / (2.0 * pi * kInsulation_safe * pipeLength_safe);

hAir_safe = max(hAir, epsilon);
Aext      = 2.0 * pi * r3_safe * pipeLength_safe;
Rconv     = 1.0 / (hAir_safe * Aext);

emiss_safe  = max(emissivitySurfacePipe, epsilon);
stefan_safe = max(stefanBoltz,           epsilon);

Tsum2 = Tfluid_safe^2 + Tamb_safe^2;
Tsum1 = Tfluid_safe   + Tamb_safe;

Rrad = 1.0 / (emiss_safe * stefan_safe * Aext * Tsum2 * Tsum1);

Rsurf_inv = (1.0 / Rconv) + (1.0 / Rrad);
Rsurf     = 1.0 / max(Rsurf_inv, epsilon);

Rtot = max(Rcond + Rsurf, epsilon);

PlossHeat_W  = max(0.0, (Tfluid_safe - Tamb_safe) / Rtot);
PlossHeat_kW = PlossHeat_W / 1000.0;

PheatDelivered = max(0.0, PheatToDemandTransport - PlossHeat_kW);

% TOTALS
DDemandTransport = PlossElec + PlossHeat_kW;

PfromDemandTransport = PheatDelivered + PelecDelivered;

end

== matlab function EST/Extraction system1/Extraction system ==
  data: PfromBattery input; PtoDemand output; DExtraction output; etaDischarge input
function [PtoDemand, DExtraction] = batteryExtraction(PfromBattery, etaDischarge)

% Battery Extraction subsystem
% Inputs and outputs are in kW.

PfromBattery = max(0.0, PfromBattery);

eta = max(0.0, min(1.0, etaDischarge));

PtoDemand   = eta * PfromBattery;
DExtraction = (1.0 - eta) * PfromBattery;

end

== matlab function EST/Injection system1/Injection system ==
  data: PtoBatteryInjection input; pFromInjection output; efficiencyBatteryCharge input; dInjection output
function [pFromInjection, dInjection] = batteryInjection(PtoBatteryInjection, efficiencyBatteryCharge)

% Battery Injection subsystem
% Inputs and outputs are in kW.

PtoBatteryInjection = max(0.0, PtoBatteryInjection);

eta = max(0.0, min(1.0, efficiencyBatteryCharge));

pFromInjection = eta * PtoBatteryInjection;
dInjection     = (1.0 - eta) * PtoBatteryInjection;

end

== matlab function EST/Storage containment system1/Storage system ==
  data: DStorage output; PtoStorage input; PfromBattery input; EStorage input; EStorageNew output
function [DStorage, EStorageNew] = BatteryStorage(PtoStorage, PfromBattery, EStorage)

% Battery Storage subsystem
% PtoStorage and PfromBattery are in kW.
% EStorage and EStorageNew are in J.

dt = 900; % [s]

PtoStorageW   = max(0.0, PtoStorage)   * 1000.0;
PfromBatteryW = max(0.0, PfromBattery) * 1000.0;

EStorageNew = EStorage + (PtoStorageW - PfromBatteryW) * dt;

EStorageNew = max(0.0, EStorageNew);

% No efficiency losses here.
% Charge loss is in batteryInjection.
% Discharge loss is in batteryExtraction.
DStorage = 0.0;

end

== matlab function EST/Injection system/Injection system ==
  data: PtoInjection input; pFromInjection output; tempTank input; dInjection output; tempEnv input; dTdt output; areaTank input; thicknessSteel input; thicknessInsulation input; kSteel input; kInsulation input; hAir input; emissivitySurface input; stefanBoltz input; efficiencyInjection input; mCpTotal input
function [pFromInjection, dInjection, dTdt] = injection(PtoInjection, tempTank, tempEnv, areaTank, thicknessSteel, thicknessInsulation, kSteel, kInsulation, hAir, emissivitySurface, stefanBoltz, efficiencyInjection, mCpTotal)

% Sorption Injection subsystem
% Power signals are in kW.
% This block only handles conversion efficiency.
% Tank temperature dynamics are handled in the Storage block.

PtoInjection = max(0.0, PtoInjection);

eta = max(0.0, min(1.0, efficiencyInjection));

pFromInjection = eta * PtoInjection;
dInjection     = (1.0 - eta) * PtoInjection;

% Temperature is not updated here anymore.
dTdt = 0.0;

end

== matlab function EST/Transport from supply/Transport from supply ==
  data: PfromSupplyTransport output; DSupplyTransport output; PtoSupplyTransport input; cableResistivity input; cableLength input; current input; cableArea input
function [PfromSupplyTransport, DSupplyTransport] = supplyTransport(PtoSupplyTransport, cableResistivity, cableLength, current, cableArea)

% Supply transport subsystem
% Input/output power signals are in kW.
% Cable loss is calculated in W, then converted to kW.

epsilon = 1e-9;

PtoSupplyTransport = max(0.0, PtoSupplyTransport);

cableArea_safe = max(cableArea, epsilon);

R = cableResistivity * (2.0 * cableLength / cableArea_safe); % [Ohm]

% Only have current/loss when there is power being transported
if PtoSupplyTransport > 0
    DSupplyTransport = (current^2 * R) / 1000.0; % [kW]
else
    DSupplyTransport = 0.0;
end

% Loss cannot exceed incoming power
DSupplyTransport = min(DSupplyTransport, PtoSupplyTransport);

PfromSupplyTransport = PtoSupplyTransport - DSupplyTransport;

end

== matlab function EST/Controller/Controller ==
  data: PdirectHeat output; PdirectElec output; PtoBatteryInjection output; PtoSorptionInjection output; PfromBattery output; PfromSorptionStorage output; Pcurtailed output; PSupply input; PDemand input; ESorption input; EBattery input; t input; EStorageMin input; EStorageMax input; EBatteryMin input; EBatteryMax input; alphaSplit input; efficiencyInjection input; efficiencyBatteryCharge input; etaBatteryDischarge input; alphaLoss input; dt input; PunmetHeat output; PunmetElec output; PmaxBatteryCharge input; PmaxBatteryDischarge input; PmaxSorptionCharge input; PmaxSorptionDischarge input
function [PdirectHeat, PdirectElec, PtoBatteryInjection, PtoSorptionInjection, PfromBattery, PfromSorptionStorage, Pcurtailed, PunmetHeat, PunmetElec] = controller(PSupply, PDemand, ESorption, EBattery, t, EStorageMin, EStorageMax, EBatteryMin, EBatteryMax, alphaSplit, efficiencyInjection, efficiencyBatteryCharge, etaBatteryDischarge, alphaLoss, dt, PmaxBatteryCharge, PmaxBatteryDischarge, PmaxSorptionCharge, PmaxSorptionDischarge)

% Controller for hybrid battery + sorption storage.
% Power signals are in kW.
% Stored energy signals are in J.
% t is simulation time in seconds.

epsilon = 1e-9;

PSupply = max(0.0, PSupply);
PDemand = max(0.0, PDemand);

dt_safe = max(dt, epsilon);

alphaSplit = max(0.0, min(1.0, alphaSplit));

etaSorptionCharge = max(epsilon, min(1.0, efficiencyInjection));
etaBatteryCharge  = max(epsilon, min(1.0, efficiencyBatteryCharge));
etaBatteryDis     = max(epsilon, min(1.0, etaBatteryDischarge));

alphaLoss = max(0.0, min(1.0, alphaLoss));
etaSorptionExtract = max(epsilon, 1.0 - alphaLoss);

% Split demand into heating and electricity
PheatDemand = alphaSplit * PDemand;
PelecDemand = (1.0 - alphaSplit) * PDemand;

% Determine day of year
dayOfYear = floor(t / 86400.0) + 1;
dayOfYear = mod(dayOfYear - 1, 365) + 1;

% Simple day/night check based on solar availability
isNight = PSupply < 0.01;

% Seasonal logic
% Charge sorption mainly from May to September.
isSorptionChargeSeason = dayOfYear >= 121 && dayOfYear <= 273;

% Use sorption for heating mainly from October to April.
isHeatingSeason = dayOfYear >= 274 || dayOfYear <= 120;

% ---------------------------------------------------------
% 1. DIRECT SUPPLY TO DEMAND FIRST
% ---------------------------------------------------------

PdirectTotal = min(PSupply, PDemand);

PdirectHeat = alphaSplit * PdirectTotal;
PdirectElec = (1.0 - alphaSplit) * PdirectTotal;

PsolarSurplus = max(0.0, PSupply - PdirectTotal);

PheatDeficit = max(0.0, PheatDemand - PdirectHeat);
PelecDeficit = max(0.0, PelecDemand - PdirectElec);

% ---------------------------------------------------------
% 2. STORAGE DISCHARGE ONLY WHEN THERE IS DEFICIT
% ---------------------------------------------------------

% Battery discharges at night for electricity only
EBatteryAvailable = max(0.0, EBattery - EBatteryMin);
PfromBatteryEnergyLimit = EBatteryAvailable / dt_safe / 1000.0;

if isNight
    PfromBatteryRequest = PelecDeficit / etaBatteryDis;
else
    PfromBatteryRequest = 0.0;
end

PfromBattery = min([PfromBatteryRequest, PfromBatteryEnergyLimit, PmaxBatteryDischarge]);

PelecFromBatteryUseful = etaBatteryDis * PfromBattery;

PunmetElec = max(0.0, PelecDeficit - PelecFromBatteryUseful);

% Sorption discharges at night during heating season for heat only
ESorptionAvailable = max(0.0, ESorption - EStorageMin);
PfromSorptionEnergyLimit = ESorptionAvailable / dt_safe / 1000.0;

if isNight && isHeatingSeason
    PfromSorptionRequest = PheatDeficit / etaSorptionExtract;
else
    PfromSorptionRequest = 0.0;
end

PfromSorptionStorage = min([PfromSorptionRequest, PfromSorptionEnergyLimit, PmaxSorptionDischarge]);

PheatFromSorptionUseful = etaSorptionExtract * PfromSorptionStorage;

PunmetHeat = max(0.0, PheatDeficit - PheatFromSorptionUseful);

% ---------------------------------------------------------
% 3. CHARGE STORAGE ONLY WITH SURPLUS
% ---------------------------------------------------------

PtoBatteryInjection = 0.0;
PtoSorptionInjection = 0.0;

% Battery gets priority because it is daily storage
EBatteryRoom = max(0.0, EBatteryMax - EBattery);
PbatteryChargeCapacity = EBatteryRoom / dt_safe / 1000.0 / etaBatteryCharge;

PtoBatteryInjection = min([PsolarSurplus, PbatteryChargeCapacity, PmaxBatteryCharge]);

PsolarSurplus = PsolarSurplus - PtoBatteryInjection;

% Sorption only charges in the charging season, slowly
if isSorptionChargeSeason
    ESorptionRoom = max(0.0, EStorageMax - ESorption);
    PsorptionChargeCapacity = ESorptionRoom / dt_safe / 1000.0 / etaSorptionCharge;

    PtoSorptionInjection = min([PsolarSurplus, PsorptionChargeCapacity, PmaxSorptionCharge]);

    PsolarSurplus = PsolarSurplus - PtoSorptionInjection;
end

% Anything left is curtailed
Pcurtailed = max(0.0, PsolarSurplus);

end
